simulink model "powerproject"  (R2023b)
settings: Solver=VariableStepAuto  StartTime=0.0  StopTime=1.0  RelTol=1e-3
libraries: spsSeriesRLCBranchLib x5, spsVoltageMeasurementLib x3, spsCurrentMeasurementLib x2, spsDCVoltageSourceLib x1, spsDiodeLib x1, spsGroundLib x1, spsMosfetLib x1, spsPWMGeneratorDCDCLib x1, sps_lib x1
settings Model: Creator=vaide  LastModifiedBy=vaide

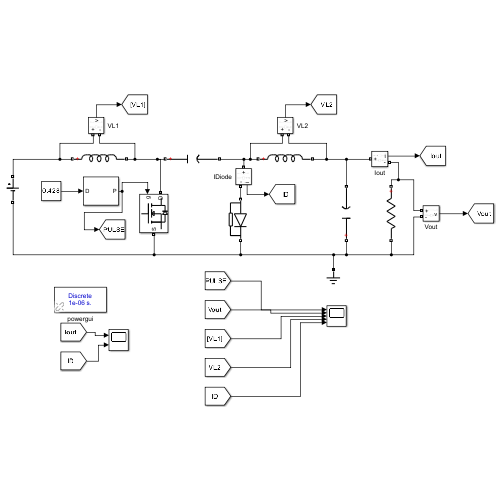
[thumbnail: Simulink's stored preview of the top-level diagram]
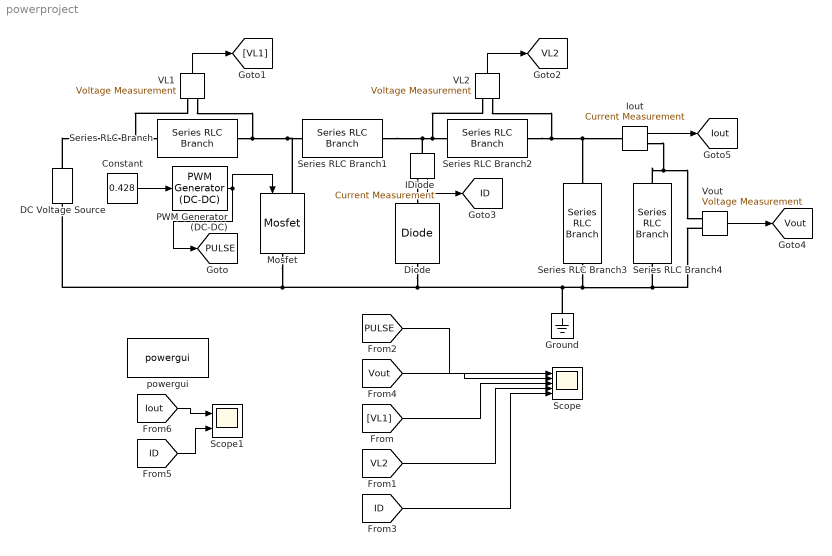
== system powerproject ==
  Constant : Constant  Value=0.428  VectorParams1D=off
  DC Voltage Source : spsDCVoltageSourceLib/DC Voltage Source  Amplitude=10  Measurements=None
  Diode : spsDiodeLib/Diode  Ron=1e-7  Lon=0  Vf=0  IC=0  UseSnubber=0  Rs=1e6  Cs=1e6  Measurements=off
  Ground : spsGroundLib/Ground  LConnTagsString=a
  IDiode : spsCurrentMeasurementLib/Current Measurement  PhasorSimulation=off  OutputType=Complex  PSBequivalent=0
  Iout : spsCurrentMeasurementLib/Current Measurement  PhasorSimulation=off  OutputType=Complex  PSBequivalent=0
  Mosfet : spsMosfetLib/Mosfet  Ron=1e-7  Lon=0  Rd=1e-10  Vfd=0  IC=0  Rs=inf  Cs=0  Measurements=off
  PWM Generator (DC-DC) : spsPWMGeneratorDCDCLib/PWM Generator (DC-DC)  Fsw=10000  Ts=0
  Scope : Scope  NumInputPorts=5
  Scope1 : Scope  NumInputPorts=2
  Series RLC Branch : spsSeriesRLCBranchLib/Series RLC Branch  LConnTagsString=__new0  RConnTagsString=__new0  BranchType=L  Resistance=0  Inductance=1e-3  SetiL0=off  InitialCurrent=0  Capacitance=0  Setx0=off  InitialVoltage=0  Measurements=None
  Series RLC Branch1 : spsSeriesRLCBranchLib/Series RLC Branch  LConnTagsString=__new0  RConnTagsString=__new0  BranchType=C  Resistance=0  Inductance=1e-3  SetiL0=off  InitialCurrent=0  Capacitance=470e-6  Setx0=off  InitialVoltage=0  Measurements=None
  Series RLC Branch2 : spsSeriesRLCBranchLib/Series RLC Branch  LConnTagsString=__new0  RConnTagsString=__new0  BranchType=L  Resistance=1  Inductance=1e-3  SetiL0=off  InitialCurrent=0  Capacitance=1e-6  Setx0=off  InitialVoltage=0  Measurements=None
  Series RLC Branch3 : spsSeriesRLCBranchLib/Series RLC Branch  LConnTagsString=__new0  RConnTagsString=__new0  BranchType=C  Resistance=1  Inductance=1e-3  SetiL0=off  InitialCurrent=0  Capacitance=470e-6  Setx0=off  InitialVoltage=0  Measurements=None
  Series RLC Branch4 : spsSeriesRLCBranchLib/Series RLC Branch  LConnTagsString=__new0  RConnTagsString=__new0  BranchType=R  Resistance=25  Inductance=1e-3  SetiL0=off  InitialCurrent=0  Capacitance=1e-6  Setx0=off  InitialVoltage=0  Measurements=None
  VL1 : spsVoltageMeasurementLib/Voltage Measurement  PhasorSimulation=off  OutputType=Complex  PSBequivalent=0
  VL2 : spsVoltageMeasurementLib/Voltage Measurement  PhasorSimulation=off  OutputType=Complex  PSBequivalent=0
  Vout : spsVoltageMeasurementLib/Voltage Measurement  PhasorSimulation=off  OutputType=Complex  PSBequivalent=0
  powergui : sps_lib/powergui  Priority=1  SimulationMode=Discrete  SampleTime=1e-6  frequency=60  Iterations=50  frequencyindice=0  Pbase=100e6  ErrMax=1e-4  UnitsV=kV  UnitsW=MW  buscounter=0  FunctionMessages=off  echomessages=off  EnableUseOfTLC=off  CurrentSourceSwitches=off  DisableSnubberDevices=off  DisableRonSwitches=off  DisableVfSwitches=off  DisplayEquations=off  AutomaticDiscreteSolvers=off  SolverType=Tustin/Backward Euler (TBE)  Interpol=off  ExternalGateDelay=off  methode=off  Ts=100  x0status=blocks  SPID=on  SwTol=0  HookPort=off  NonlinearTolerance=1e-4  nMaxIteration=100  ContinueOnMaxIteration=off  RestoreLinks=warning  ResistiveCurrentMeasurement=off  Frange=[0:2:500]  Ylog=off  Xlog=on  ShowGrid=off  save=off  variable=ZData  structure=0  ZoomFFT=off  StartTime=0.0  cycles=1  DisplayStyle=1  fundamental=60  FreqAxis=off  MaxFrequency=1000  frequencyindicesteady=1  RmsSteady=1  display=off
  tag scope: ID=global, Iout=global, PULSE=global, VL2=global, Vout=global
  wires:
  Constant/1 -> PWM Generator (DC-DC)/1
  IDiode/1 -> [ID]
  PWM Generator (DC-DC)/1 -> [PULSE], Mosfet/1
  VL1/1 -> [VL1]
  VL2/1 -> [VL2]
  Vout/1 -> [Vout]
  [PULSE] -> Scope/1
  [Vout] -> Scope/2
  [VL1] -> Scope/3
  [VL2] -> Scope/4
  [ID] -> Scope/5
  Iout/1 -> [Iout]
  [Iout] -> Scope1/1
  [ID] -> Scope1/2
  connections:
  DC Voltage Source/RConn1 -- VL1/LConn1 -- Series RLC Branch/LConn1
  Series RLC Branch/RConn1 -- VL1/LConn2 -- Mosfet/LConn1 -- Series RLC Branch1/LConn1
  Series RLC Branch1/RConn1 -- IDiode/LConn1 -- VL2/LConn1 -- Series RLC Branch2/LConn1
  IDiode/RConn1 -- Diode/LConn1
  Series RLC Branch4/LConn1 -- Iout/RConn1 -- Vout/LConn1
  Series RLC Branch3/LConn1 -- Ground/LConn1 -- Diode/RConn1 -- Mosfet/RConn1 -- DC Voltage Source/LConn1 -- Vout/LConn2 -- Series RLC Branch4/RConn1
  Series RLC Branch2/RConn1 -- Iout/LConn1 -- Series RLC Branch3/RConn1 -- VL2/LConn2
